simulink model "proportionalNav_withControlSystem"  (R2023b)
settings: Solver=ode4  StartTime=0.0  StopTime=inf  FixedStep=0.001  RelTol=1e-3
model workspace: external: MAT-File C:\proj\simulink_runner.mat (data not in the file)
values from neighbouring files (symbols this model uses):
  Beta = X(5)    [matlab_control_with_comment.m]
  coef_data = struct()    [matlab_control_with_comment.m]
  dry_mass = missile.dry_mass    [matlab_control_with_comment.m]
  fuel_mass = current_fuel_mass + fuel_structure_mass    [matlab_control_with_comment.m]
  g = 9.81    [matlab_control_with_comment.m]
  lref = missile.lref    [matlab_control_with_comment.m]
  q = X_s(11)    [matlab_control_with_comment.m]
  R_Mx = X(6)    [matlab_control_with_comment.m]
  R_Mz = X(7)    [matlab_control_with_comment.m]
  R_Tx = X(1)    [matlab_control_with_comment.m]
  R_Tz = X(2)    [matlab_control_with_comment.m]
  S = missile.S    [matlab_control_with_comment.m]
  t_b = thrust.t_b    [matlab_control_with_comment.m]
  T_total = thrust.T_total    [matlab_control_with_comment.m]
  theta = X(10)    [matlab_control_with_comment.m]
  V_Mx = X(8)    [matlab_control_with_comment.m]
  V_Mz = X(9)    [matlab_control_with_comment.m]
  V_T = target.V_T    [matlab_control_with_comment.m]
  XNP = missile.XNP    [matlab_control_with_comment.m]
  XNT = target.XNT    [matlab_control_with_comment.m]
libraries: simulink_extras x3, simulink x2
settings Model: NumberOfSteps=15  Creator=hamdi  LastModifiedBy=furkan
settings SolverCC: InitialStep=0.001  ZeroCrossAlgorithm=Adaptive

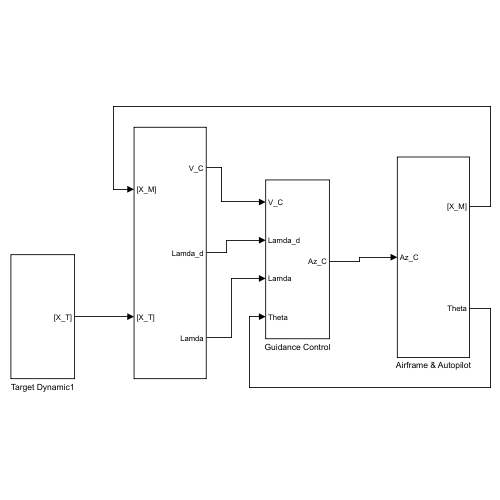
[thumbnail: Simulink's stored preview of the top-level diagram]
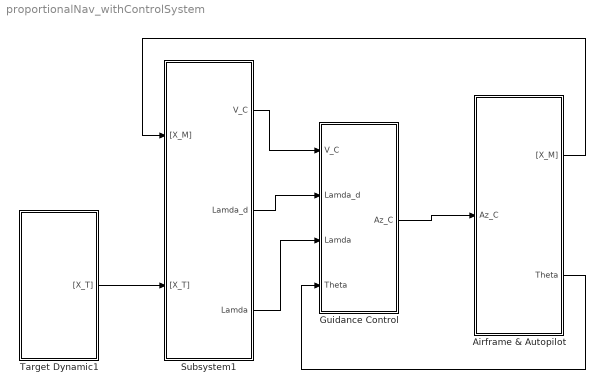
== system proportionalNav_withControlSystem ==
  Airframe & Autopilot : Subsystem
  Guidance Control : Subsystem
  Subsystem1 : Subsystem
  Target Dynamic1 : Subsystem
  wires:
  Subsystem1/2(Lamda_d) -> Guidance Control/2(Lamda_d)
  Target Dynamic1/1("[X_T]") -> Subsystem1/2("[X_T]")
  Subsystem1/1(V_C) -> Guidance Control/1(V_C)
  Subsystem1/3(Lamda) -> Guidance Control/3(Lamda)
  Guidance Control/1(Az_C) -> Airframe & Autopilot/1(Az_C)
  Airframe & Autopilot/1("[X_M]") -> Subsystem1/1("[X_M]")
  Airframe & Autopilot/2(Theta) -> Guidance Control/4(Theta)

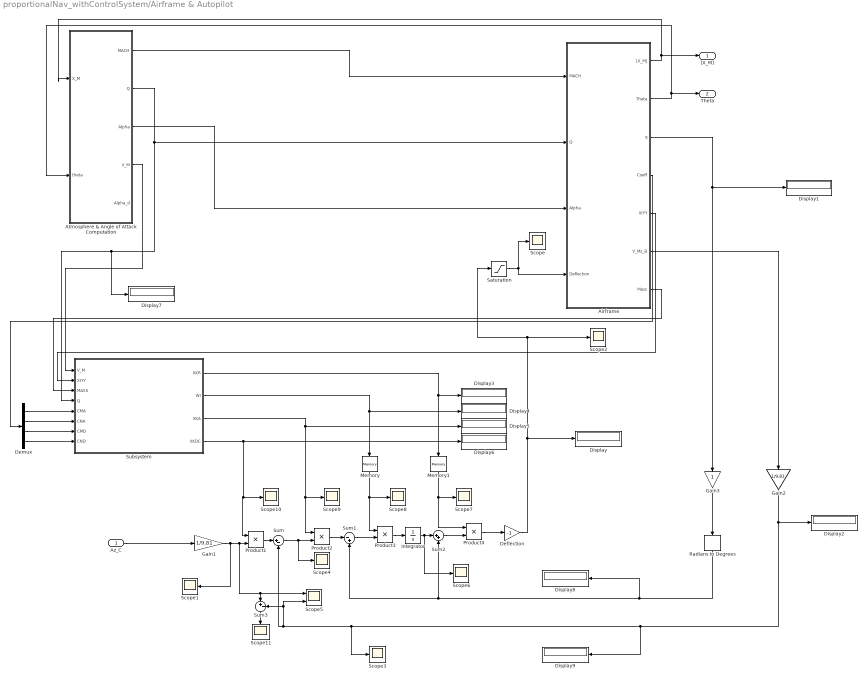
== system proportionalNav_withControlSystem/Airframe & Autopilot ==
  Az_C : Inport
  Airframe : Subsystem
  Atmosphere & Angle of Attack Computation : Subsystem
  Deflection : Gain  Gain=-1
  Demux : Demux
  Display{,1..9} (10 alike) : Display
  Gain1 : Gain  Gain=1/9.81
  Gain2 : Gain  Gain=1/9.81
  Gain3 : Gain
  Integrator : Integrator
  Memory : Memory
  Memory1 : Memory
  Product{1..4} (4 alike) : Product
  Radians to Degrees : simulink_extras/Transformations/Radians to Degrees
  Saturation : Saturate  UpperLimit=19  LowerLimit=-19
  Scope{,1..4,6..11} (11 alike) : Scope
  Scope5 : Scope  NumInputPorts=2
  Subsystem : Subsystem
  Sum : Sum  Inputs=|+-
  Sum1 : Sum  Inputs=|-+
  Sum2 : Sum  Inputs=|++
  Sum3 : Sum  Inputs=|+-
  "[X_M]" : Outport
  Theta : Outport  Port=2
  wires:
  Atmosphere & Angle of Attack Computation/1(MACH) -> Airframe/1(MACH)
  Atmosphere & Angle of Attack Computation/3(Alpha) -> Airframe/3(Alpha)
  Airframe/1("[X_M]") -> "[X_M]"/1, Atmosphere & Angle of Attack Computation/1(X_M)
  Airframe/2(Theta) -> Theta/1, Atmosphere & Angle of Attack Computation/2(theta)
  Product2/1 -> Sum1/1
  Product1/1 -> Sum/1
  Product3/1 -> Integrator/1
  Sum/1 -> Scope4/1, Product2/2
  Sum1/1 -> Product3/2
  Sum2/1 -> Product4/2
  Product4/1 -> Deflection/1
  Subsystem/1(XKR) -> Display3/1, Memory1/1
  Atmosphere & Angle of Attack Computation/4(V_M) -> Subsystem/1(V_M)
  Airframe/4(Coeff) -> Demux/1
  Demux/1 -> Subsystem/5(CMA)
  Demux/2 -> Subsystem/6(CNA)
  Demux/3 -> Subsystem/7(CMD)
  Demux/4 -> Subsystem/8(CND)
  Airframe/5(XIYY) -> Subsystem/2(XIYY)
  Airframe/7(Mass) -> Subsystem/3(MASS)
  Subsystem/2(WI) -> Display4/1, Memory/1
  Memory/1 -> Scope8/1, Product3/1
  Memory1/1 -> Scope7/1, Product4/1
  Integrator/1 -> Scope6/1, Sum2/1
  Gain3/1 -> Radians to Degrees/1
  Deflection/1 -> Saturation/1, Scope2/1, Display/1
  Radians to Degrees/1 -> Display8/1, Sum2/2, Sum1/2
  Atmosphere & Angle of Attack Computation/2(Q) -> Subsystem/4(Q), Display7/1, Airframe/2(Q)
  Airframe/3(q) -> Gain3/1, Display1/1
  Airframe/6(V_Mz_B) -> Gain2/1
  Gain1/1 -> Scope1/1, Sum3/1, Scope5/1, Product1/2
  Saturation/1 -> Scope/1, Airframe/4(Deflection)
  Subsystem/4(XKDC) -> Product1/1, Scope10/1, Display6/1
  Subsystem/3(XKA) -> Scope9/1, Product2/1, Display5/1
  Gain2/1 -> Display2/1, Display9/1, Sum3/2, Scope5/2, Sum/2, Scope3/1
  Sum3/1 -> Scope11/1
  Az_C/1 -> Gain1/1

== system proportionalNav_withControlSystem/Guidance Control ==
  V_C : Inport
  Lamda_d : Inport  Port=2
  Lamda : Inport  Port=3
  Theta : Inport  Port=4
  Cos : Trigonometry  Operator=cos
  Display : Display
  Display1 : Display
  Display2 : Display
  "Effective Navigation Ratio " : Constant  Value=XNP
  Gain1 : Gain  Gain=1/g
  Product : Product
  Product9 : Product  Inputs=3
  Scope1 : Scope
  Subtract : Sum  Inputs=+-
  Az_C : Outport
  wires:
  V_C/1 -> Display/1, Product9/3
  "Effective Navigation Ratio "/1 -> Product9/1
  Lamda_d/1 -> Display1/1, Product9/2
  Product9/1 -> Az_C/1, Product/1, Gain1/1
  Gain1/1 -> Scope1/1, Display2/1
  Theta/1 -> Subtract/1
  Subtract/1 -> Cos/1
  Cos/1 -> Product/2
  Lamda/1 -> Subtract/2

== system proportionalNav_withControlSystem/Subsystem1 ==
  "[X_M]" : Inport
  "[X_T]" : Inport  Port=2
  Compare To Zero : simulink/Logic and Bit Operations/Compare To Zero  relop=<=  OutDataTypeStr=boolean
  Demux : Demux
  Demux1 : Demux
  Display : Display
  Scope : Scope
  Scope2 : Scope
  Stop Simulation : Stop
  Subsystem2 : Subsystem
  V_C : Outport
  Lamda_d : Outport  Port=2
  Lamda : Outport  Port=3
  wires:
  "[X_T]"/1 -> Demux/1
  "[X_M]"/1 -> Demux1/1
  Subsystem2/2(Lamda_d) -> Scope2/1, Lamda_d/1
  Subsystem2/1(V_C) -> Compare To Zero/1, V_C/1, Display/1, Scope/1
  Demux1/1 -> Subsystem2/1(R_Mx)  "R_Mx"
  Demux1/2 -> Subsystem2/2(R_Mz)  "R_Mz"
  Demux1/3 -> Subsystem2/3(V_Mx)  "V_Mx"
  Demux1/4 -> Subsystem2/4(V_Mz)  "V_Mz"
  Demux/1 -> Subsystem2/5(R_Tx)  "R_Tx"
  Demux/2 -> Subsystem2/6(R_Tz)  "R_Tz"
  Demux/3 -> Subsystem2/7(V_Tx)  "V_Tx"
  Demux/4 -> Subsystem2/8(V_Tz)  "V_Tz"
  Compare To Zero/1 -> Stop Simulation/1
  Subsystem2/4(Lamda) -> Lamda/1

== system proportionalNav_withControlSystem/Target Dynamic1 ==
  Mux : Mux
  Subsystem : Subsystem
  "[X_T]" : Outport
  wires:
  Mux/1 -> "[X_T]"/1
  Subsystem/1(R_Tx) -> Mux/1
  Subsystem/2(R_Tz) -> Mux/2
  Subsystem/3(V_Tx) -> Mux/3
  Subsystem/4(V_Tz) -> Mux/4

== system proportionalNav_withControlSystem/Airframe & Autopilot/Airframe ==
  MACH : Inport
  Q : Inport  Port=2
  Alpha : Inport  Port=3
  Deflection : Inport  Port=4
  Acceleration Calculation : Subsystem
  Aerodynamic : Subsystem
  Integration : Subsystem
  Thrust : Subsystem
  "[X_M]" : Outport
  Theta : Outport  Port=2
  q : Outport  Port=3
  Coeff : Outport  Port=4
  XIYY : Outport  Port=5
  V_Mz_B : Outport  Port=6
  Mass : Outport  Port=7
  wires:
  MACH/1 -> Aerodynamic/2(MACH)
  Q/1 -> Aerodynamic/3(Q)
  Alpha/1 -> Aerodynamic/4(Alpha)
  Deflection/1 -> Aerodynamic/5(Deflection)
  Integration/1("[X_M]") -> "[X_M]"/1
  Aerodynamic/1(Aero_X_force) -> Acceleration Calculation/4(Aero_X_force)
  Thrust/1(Thrust) -> Acceleration Calculation/2(Thrust)
  Thrust/3(xcg) -> Aerodynamic/1(XCG)
  Thrust/2(Mass) -> Mass/1, Acceleration Calculation/3(Mass)
  Aerodynamic/3(Moment) -> Integration/3(Moment)
  Acceleration Calculation/1(A_Mx_I) -> Integration/1(A_Mx)
  Acceleration Calculation/2(A_Mz_I) -> Integration/2(A_Mz)
  Thrust/4(Iyy) -> XIYY/1, Integration/4(Iyy)
  Integration/3(q) -> q/1
  Integration/2(Theta) -> Theta/1, Acceleration Calculation/1(Theta)
  Aerodynamic/4(Coeff) -> Coeff/1
  Aerodynamic/2(Aero_Z_force) -> Acceleration Calculation/5(Aero_Z_force)
  Acceleration Calculation/3(Out3) -> V_Mz_B/1

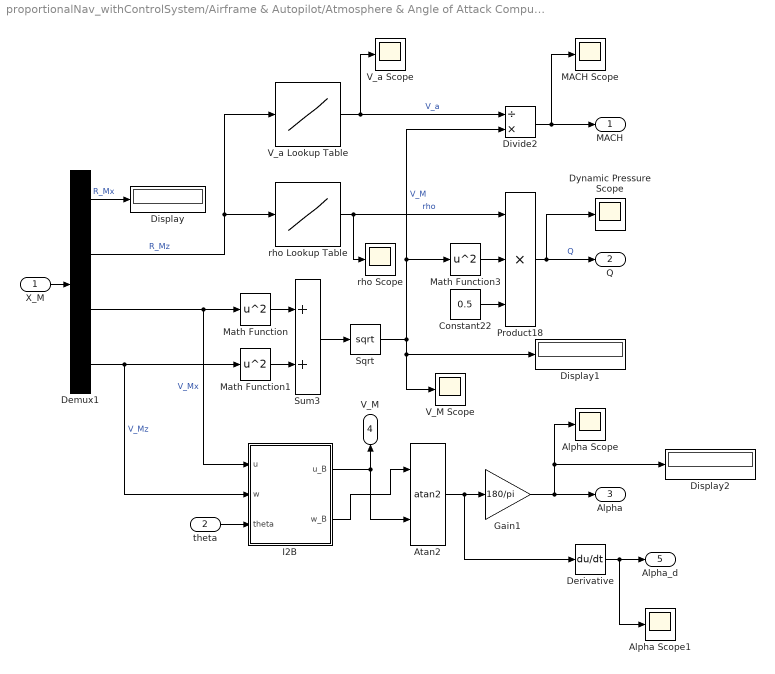
== system proportionalNav_withControlSystem/Airframe & Autopilot/Atmosphere & Angle of Attack Computation ==
  X_M : Inport
  theta : Inport  Port=2
  Alpha Scope : Scope
  Alpha Scope1 : Scope
  Atan2 : Trigonometry  Operator=atan2
  Constant22 : Constant  Value=0.5
  Demux1 : Demux
  Derivative : Derivative
  Display : Display
  Display1 : Display
  Display2 : Display
  Divide2 : Product  Inputs=/*
  Dynamic Pressure Scope : Scope
  Gain1 : Gain  Gain=180/pi
  I2B : MATLAB Function  TreatAsAtomicUnit=on
  MACH Scope : Scope
  Math Function : Math  Operator=square
  Math Function1 : Math  Operator=square
  Math Function3 : Math  Operator=square
  Product18 : Product  Inputs=3
  Sqrt : Sqrt
  Sum3 : Sum
  V_M Scope : Scope
  V_a Lookup Table : Lookup_n-D  NumberOfTableDimensions=1  BreakpointsForDimension1=coef_data.alt_table  Table=coef_data.V_a_table  InternalRulePriority=Speed  RndMeth=Simplest
  V_a Scope : Scope
  rho Lookup Table : Lookup_n-D  NumberOfTableDimensions=1  BreakpointsForDimension1=coef_data.alt_table  Table=coef_data.rho_table  InternalRulePriority=Speed  RndMeth=Simplest
  rho Scope : Scope
  MACH : Outport
  Q : Outport  Port=2
  Alpha : Outport  Port=3
  V_M : Outport  Port=4
  Alpha_d : Outport  Port=5
  wires:
  Demux1/3 -> I2B/1(u), Math Function/1  "V_Mx"
  Demux1/1 -> Display/1  "R_Mx"
  Demux1/2 -> V_a Lookup Table/1, rho Lookup Table/1  "R_Mz"
  Demux1/4 -> Math Function1/1, I2B/2(w)  "V_Mz"
  X_M/1 -> Demux1/1
  Sum3/1 -> Sqrt/1
  Math Function1/1 -> Sum3/2
  Math Function/1 -> Sum3/1
  Math Function3/1 -> Product18/2
  Sqrt/1 -> Display1/1, V_M Scope/1, Divide2/2, Math Function3/1  "V_M"
  Constant22/1 -> Product18/3
  Product18/1 -> Q/1, Dynamic Pressure Scope/1  "Q"
  rho Lookup Table/1 -> rho Scope/1, Product18/1  "rho"
  Divide2/1 -> MACH/1, MACH Scope/1
  I2B/1(u_B) -> V_M/1, Atan2/2
  I2B/2(w_B) -> Atan2/1
  theta/1 -> I2B/3(theta)
  Gain1/1 -> Alpha/1, Display2/1, Alpha Scope/1
  Atan2/1 -> Derivative/1, Gain1/1
  V_a Lookup Table/1 -> V_a Scope/1, Divide2/1  "V_a"
  Derivative/1 -> Alpha Scope1/1, Alpha_d/1

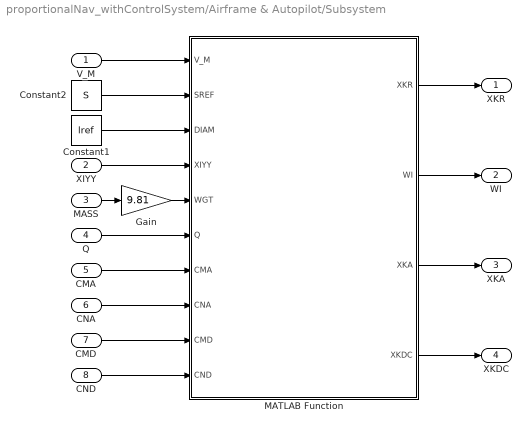
== system proportionalNav_withControlSystem/Airframe & Autopilot/Subsystem ==
  V_M : Inport
  XIYY : Inport  Port=2
  MASS : Inport  Port=3
  Q : Inport  Port=4
  CMA : Inport  Port=5
  CNA : Inport  Port=6
  CMD : Inport  Port=7
  CND : Inport  Port=8
  Constant1 : Constant  Value=lref
  Constant2 : Constant  Value=S
  Gain : Gain  Gain=9.81
  MATLAB Function : MATLAB Function  TreatAsAtomicUnit=on
  XKR : Outport
  WI : Outport  Port=2
  XKA : Outport  Port=3
  XKDC : Outport  Port=4
  wires:
  V_M/1 -> MATLAB Function/1(V_M)
  CMA/1 -> MATLAB Function/7(CMA)
  CNA/1 -> MATLAB Function/8(CNA)
  CMD/1 -> MATLAB Function/9(CMD)
  CND/1 -> MATLAB Function/10(CND)
  MATLAB Function/1(XKR) -> XKR/1
  MATLAB Function/2(WI) -> WI/1
  MATLAB Function/3(XKA) -> XKA/1
  MATLAB Function/4(XKDC) -> XKDC/1
  Q/1 -> MATLAB Function/6(Q)
  Constant2/1 -> MATLAB Function/2(SREF)
  Constant1/1 -> MATLAB Function/3(DIAM)
  XIYY/1 -> MATLAB Function/4(XIYY)
  MASS/1 -> Gain/1
  Gain/1 -> MATLAB Function/5(WGT)

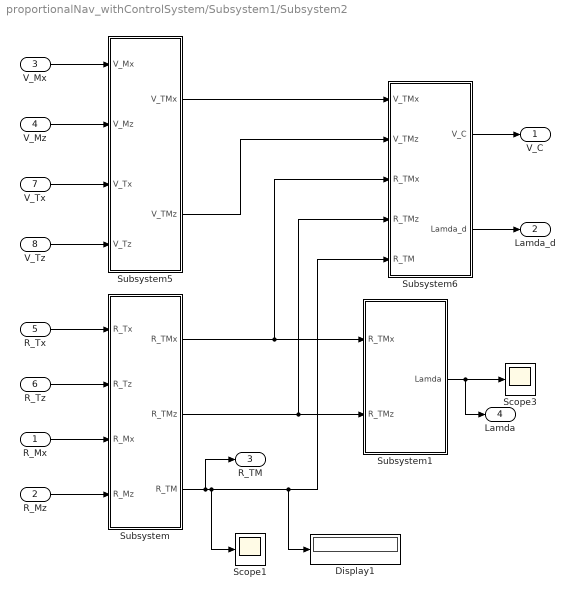
== system proportionalNav_withControlSystem/Subsystem1/Subsystem2 ==
  R_Mx : Inport
  R_Mz : Inport  Port=2
  V_Mx : Inport  Port=3
  V_Mz : Inport  Port=4
  R_Tx : Inport  Port=5
  R_Tz : Inport  Port=6
  V_Tx : Inport  Port=7
  V_Tz : Inport  Port=8
  Display1 : Display
  Scope1 : Scope
  Scope3 : Scope
  Subsystem : Subsystem
  Subsystem1 : Subsystem
  Subsystem5 : Subsystem
  Subsystem6 : Subsystem
  V_C : Outport
  Lamda_d : Outport  Port=2
  R_TM : Outport  Port=3
  Lamda : Outport  Port=4
  wires:
  Subsystem/2(R_TMz) -> Subsystem6/4(R_TMz), Subsystem1/2(R_TMz)
  Subsystem1/1(Lamda) -> Lamda/1, Scope3/1
  Subsystem5/1(V_TMx) -> Subsystem6/1(V_TMx)
  Subsystem/3(R_TM) -> R_TM/1, Subsystem6/5(R_TM), Display1/1, Scope1/1
  V_Tz/1 -> Subsystem5/4(V_Tz)
  Subsystem5/2(V_TMz) -> Subsystem6/2(V_TMz)
  Subsystem/1(R_TMx) -> Subsystem6/3(R_TMx), Subsystem1/1(R_TMx)
  V_Tx/1 -> Subsystem5/3(V_Tx)
  V_Mz/1 -> Subsystem5/2(V_Mz)
  Subsystem6/1(V_C) -> V_C/1
  Subsystem6/2(Lamda_d) -> Lamda_d/1
  V_Mx/1 -> Subsystem5/1(V_Mx)
  R_Mz/1 -> Subsystem/4(R_Mz)
  R_Tx/1 -> Subsystem/1(R_Tx)
  R_Mx/1 -> Subsystem/3(R_Mx)
  R_Tz/1 -> Subsystem/2(R_Tz)

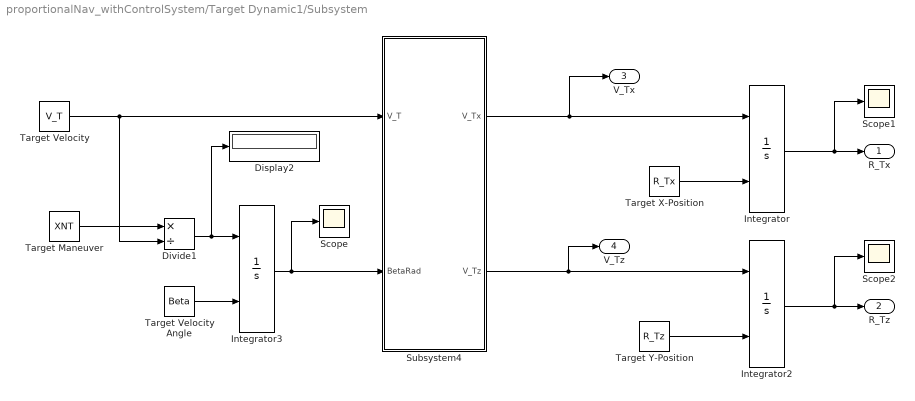
== system proportionalNav_withControlSystem/Target Dynamic1/Subsystem ==
  Display2 : Display
  Divide1 : Product  Inputs=*/
  Integrator : Integrator  InitialConditionSource=external
  Integrator2 : Integrator  InitialConditionSource=external
  Integrator3 : Integrator  InitialConditionSource=external
  Scope : Scope
  Scope1 : Scope
  Scope2 : Scope
  Subsystem4 : Subsystem
  Target Maneuver : Constant  Value=XNT
  Target Velocity : Constant  Value=V_T
  Target Velocity Angle : Constant  Value=Beta
  "Target X-Position " : Constant  Value=R_Tx
  "Target Y-Position " : Constant  Value=R_Tz
  R_Tx : Outport
  R_Tz : Outport  Port=2
  V_Tx : Outport  Port=3
  V_Tz : Outport  Port=4
  wires:
  Target Velocity/1 -> Divide1/2, Subsystem4/1(V_T)
  Subsystem4/2(V_Tz) -> V_Tz/1, Integrator2/1
  Subsystem4/1(V_Tx) -> V_Tx/1, Integrator/1
  Integrator3/1 -> Subsystem4/2(BetaRad), Scope/1
  Integrator/1 -> Scope1/1, R_Tx/1
  "Target Y-Position "/1 -> Integrator2/2
  "Target X-Position "/1 -> Integrator/2
  Integrator2/1 -> R_Tz/1, Scope2/1
  Target Maneuver/1 -> Divide1/1
  Divide1/1 -> Display2/1, Integrator3/1
  Target Velocity Angle/1 -> Integrator3/2

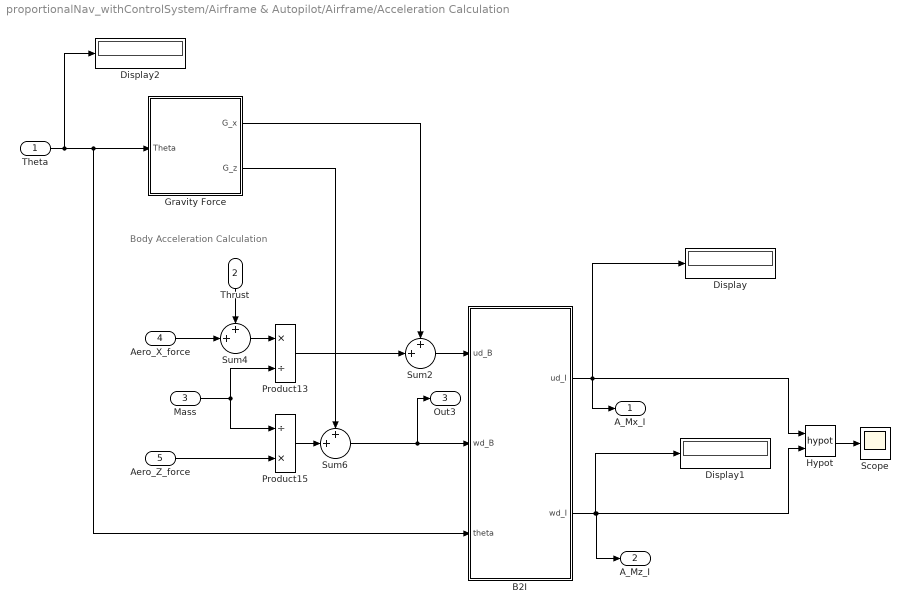
== system proportionalNav_withControlSystem/Airframe & Autopilot/Airframe/Acceleration Calculation ==
  note: Body Acceleration Calculation
  Theta : Inport
  Thrust : Inport  Port=2
  Mass : Inport  Port=3
  Aero_X_force : Inport  Port=4
  Aero_Z_force : Inport  Port=5
  B2I : MATLAB Function  TreatAsAtomicUnit=on
  Display : Display
  Display1 : Display
  Display2 : Display
  Gravity Force : Subsystem
  Hypot : Math  Operator=hypot
  Product13 : Product  Inputs=*/
  Product15 : Product  Inputs=/*
  Scope : Scope
  Sum2 : Sum  Inputs=++|
  Sum4 : Sum  Inputs=++|
  Sum6 : Sum  Inputs=++|
  A_Mx_I : Outport
  A_Mz_I : Outport  Port=2
  Out3 : Outport  Port=3
  wires:
  Theta/1 -> Display2/1, Gravity Force/1(Theta), B2I/3(theta)
  B2I/2(wd_I) -> Display1/1, Hypot/2, A_Mz_I/1
  B2I/1(ud_I) -> Hypot/1, A_Mx_I/1, Display/1
  Sum2/1 -> B2I/1(ud_B)
  Sum4/1 -> Product13/1
  Mass/1 -> Product13/2, Product15/1
  Sum6/1 -> Out3/1, B2I/2(wd_B)
  Aero_X_force/1 -> Sum4/2
  Thrust/1 -> Sum4/1
  Gravity Force/1(G_x) -> Sum2/1
  Aero_Z_force/1 -> Product15/2
  Gravity Force/2(G_z) -> Sum6/1
  Product15/1 -> Sum6/2
  Product13/1 -> Sum2/2
  Hypot/1 -> Scope/1

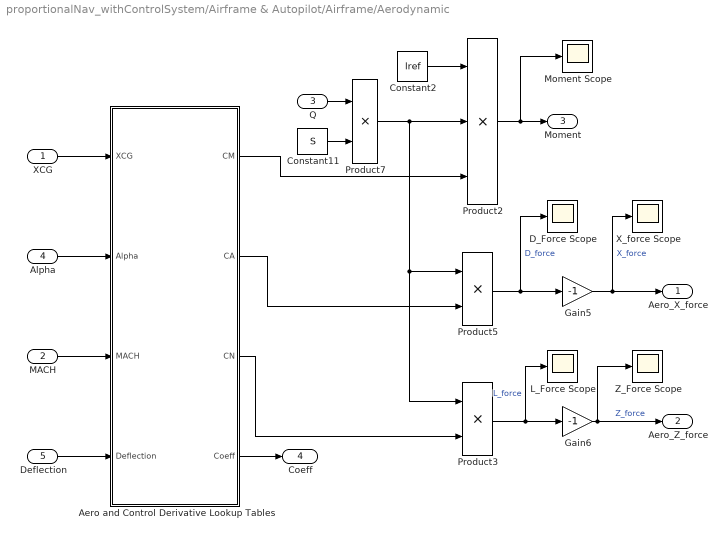
== system proportionalNav_withControlSystem/Airframe & Autopilot/Airframe/Aerodynamic ==
  XCG : Inport
  MACH : Inport  Port=2
  Q : Inport  Port=3
  Alpha : Inport  Port=4
  Deflection : Inport  Port=5
  Aero and Control Derivative Lookup Tables : Subsystem
  Constant11 : Constant  Value=S
  Constant2 : Constant  Value=lref
  D_Force Scope : Scope
  Gain5 : Gain  Gain=-1
  Gain6 : Gain  Gain=-1
  L_Force Scope : Scope
  Moment Scope : Scope
  Product2 : Product  Inputs=3
  Product3 : Product
  Product5 : Product
  Product7 : Product
  X_force Scope : Scope
  Z_Force Scope : Scope
  Aero_X_force : Outport
  Aero_Z_force : Outport  Port=2
  Moment : Outport  Port=3
  Coeff : Outport  Port=4
  wires:
  Constant11/1 -> Product7/2
  Gain6/1 -> Aero_Z_force/1, Z_Force Scope/1  "Z_force"
  Product7/1 -> Product2/2, Product3/1, Product5/1
  Product3/1 -> L_Force Scope/1, Gain6/1  "L_force"
  Product5/1 -> Gain5/1, D_Force Scope/1  "D_force"
  Gain5/1 -> Aero_X_force/1, X_force Scope/1  "X_force"
  XCG/1 -> Aero and Control Derivative Lookup Tables/1(XCG)
  Alpha/1 -> Aero and Control Derivative Lookup Tables/2(Alpha)
  MACH/1 -> Aero and Control Derivative Lookup Tables/3(MACH)
  Aero and Control Derivative Lookup Tables/1(CM) -> Product2/3
  Q/1 -> Product7/1
  Constant2/1 -> Product2/1
  Product2/1 -> Moment Scope/1, Moment/1
  Deflection/1 -> Aero and Control Derivative Lookup Tables/4(Deflection)
  Aero and Control Derivative Lookup Tables/2(CA) -> Product5/2
  Aero and Control Derivative Lookup Tables/3(CN) -> Product3/2
  Aero and Control Derivative Lookup Tables/4(Coeff) -> Coeff/1

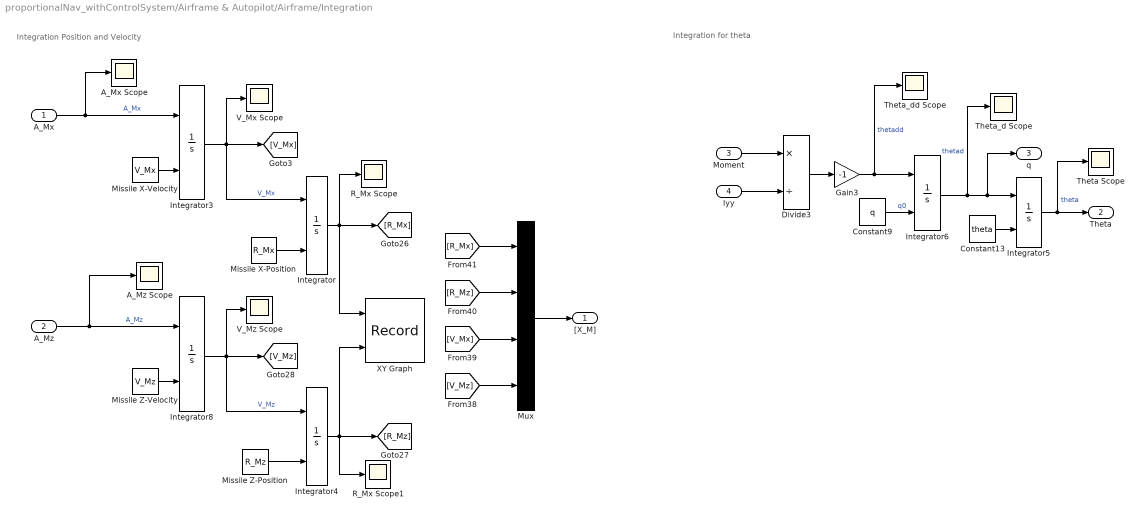
== system proportionalNav_withControlSystem/Airframe & Autopilot/Airframe/Integration ==
  note: Integration for theta
  note: Integration Position and Velocity
  A_Mx : Inport
  A_Mz : Inport  Port=2
  Moment : Inport  Port=3
  Iyy : Inport  Port=4
  A_Mx Scope : Scope
  A_Mz Scope : Scope
  Constant13 : Constant  Value=theta
  Constant9 : Constant  Value=q
  Divide3 : Product  Inputs=*/
  Gain3 : Gain  Gain=-1
  Integrator{,3..6,8} (6 alike) : Integrator  InitialConditionSource=external
  "Missile X-Position " : Constant  Value=R_Mx
  Missile X-Velocity : Constant  Value=V_Mx
  Missile Z-Position : Constant  Value=R_Mz
  Missile Z-Velocity : Constant  Value=V_Mz
  Mux : Mux
  R_Mx Scope : Scope
  R_Mx Scope1 : Scope
  Theta Scope : Scope
  Theta_d Scope : Scope
  Theta_dd Scope : Scope
  V_Mx Scope : Scope
  V_Mz Scope : Scope
  XY Graph : Record  FileSettingsInternal="{\"entries\":[{\"content\":{\"excelSettings\":{\"content\":{},\"type\":\"Streamout.ExcelSettings\"}},\"type\":\"Streamout.FileSettingStorage\",\"uuid\":\"\"}],\"packageUris\":[\"http:\\/\\/schema.mathworks.com\\/mf0\\/streamout_blocks\\/R2020a\"],\"version\":\"1.0\"}"  Layout=[1 1]  SignalsInternal="{\"entries\":[{\"content\":{\"signals\":[{\"content\":{\"blockPath\":[],\"dimensions\":[1],\"domain\":\"\",\"lineColor\":\"#a2142f\",\"plots\":[ 1 ],\"port\":1,\"sid\":[\"\"],\"signalID\":1,\"signalName\":\"Integrator\"},\"type\":\"RecordBlkView.Signal\",\"uuid\":\"\"},{\"content\":{\"blockPath\":[],\"dimensions\":[1],\"domain\":\"\",\"lineColor\":\"#139fff\",\"plots\":[ 1 ],\"port\":2,\"sid\":[\"\"],\"signalID\":2,\"signalName\":\"Integrator4\"},\"type\":\"RecordBlkView.Signal\",\"uuid\":\"\"}]},\"type\":\"RecordBlkView.InputSignals\",\"uuid\":\"\"}],\"packageUris\":[\"http:\\/\\/schema.mathworks.com\\/mf0\\/streamout_blocks\\/R2020a\"],\"version\":\"1.0\"}"  VisualizationBindings="{\"xyplotplugin\":{\"info\":[{\"series\":[{\"bindingParametersList\":[{\"parameter\":\"X-Axis\",\"signalID\":1,\"signalName\":\"Integrator\"},{\"parameter\":\"Y-Axis\",\"signalID\":2,\"signalName\":\"Integrator4\"}],\"seriesID\":0}],\"subplotID\":1}]}}"  CompatibilityTag=XY
  "[X_M]" : Outport
  Theta : Outport  Port=2
  q : Outport  Port=3
  wires:
  Constant13/1 -> Integrator5/2
  Integrator6/1 -> Theta_d Scope/1, q/1, Integrator5/1  "thetad"
  Constant9/1 -> Integrator6/2  "q0"
  Divide3/1 -> Gain3/1
  Integrator5/1 -> Theta/1, Theta Scope/1  "theta"
  Gain3/1 -> Theta_dd Scope/1, Integrator6/1  "thetadd"
  [R_Mz] -> Mux/2
  Missile Z-Velocity/1 -> Integrator8/2
  [V_Mz] -> Mux/4
  Missile Z-Position/1 -> Integrator4/2
  Integrator4/1 -> R_Mx Scope1/1, XY Graph/2, [R_Mz]
  Integrator3/1 -> [V_Mx], Integrator/1, V_Mx Scope/1  "V_Mx"
  [R_Mx] -> Mux/1
  Missile X-Velocity/1 -> Integrator3/2
  Integrator/1 -> XY Graph/1, [R_Mx], R_Mx Scope/1
  A_Mz/1 -> Integrator8/1, A_Mz Scope/1  "A_Mz"
  [V_Mx] -> Mux/3
  "Missile X-Position "/1 -> Integrator/2
  Integrator8/1 -> [V_Mz], Integrator4/1, V_Mz Scope/1  "V_Mz"
  Iyy/1 -> Divide3/2
  Moment/1 -> Divide3/1
  A_Mx/1 -> A_Mx Scope/1, Integrator3/1  "A_Mx"
  Mux/1 -> "[X_M]"/1

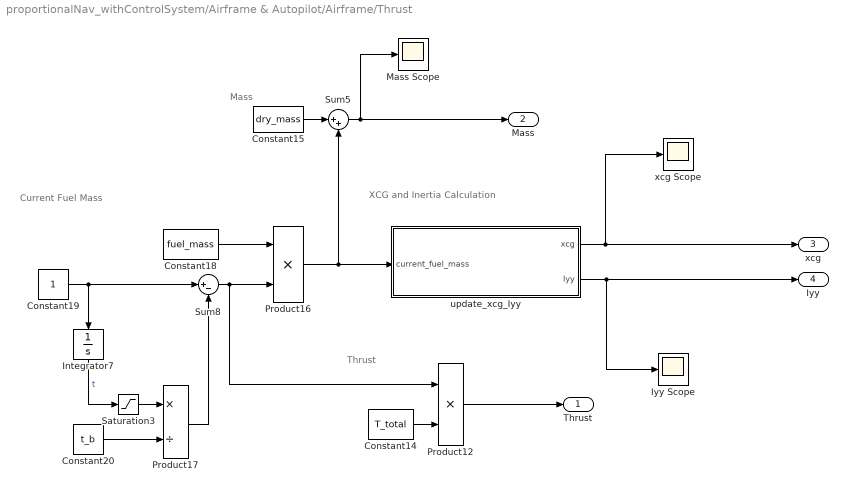
== system proportionalNav_withControlSystem/Airframe & Autopilot/Airframe/Thrust ==
  note: XCG and Inertia Calculation
  note: Mass
  note: Current Fuel Mass
  note: Thrust
  Constant14 : Constant  Value=T_total
  Constant15 : Constant  Value=dry_mass
  Constant18 : Constant  Value=fuel_mass
  Constant19 : Constant
  Constant20 : Constant  Value=t_b
  Integrator7 : Integrator
  Iyy Scope : Scope
  Mass Scope : Scope
  Product12 : Product
  Product16 : Product
  Product17 : Product  Inputs=*/
  Saturation3 : Saturate  UpperLimit=t_b  LowerLimit=0
  Sum5 : Sum  Inputs=|++
  Sum8 : Sum  Inputs=|+-
  update_xcg_Iyy : MATLAB Function  TreatAsAtomicUnit=on
  xcg Scope : Scope
  Thrust : Outport
  Mass : Outport  Port=2
  xcg : Outport  Port=3
  Iyy : Outport  Port=4
  wires:
  Constant15/1 -> Sum5/1
  Integrator7/1 -> Saturation3/1  "t"
  Saturation3/1 -> Product17/1
  Product17/1 -> Sum8/2
  Constant20/1 -> Product17/2
  Constant19/1 -> Integrator7/1, Sum8/1
  Sum8/1 -> Product12/1, Product16/2
  Constant18/1 -> Product16/1
  Product16/1 -> Sum5/2, update_xcg_Iyy/1(current_fuel_mass)
  Constant14/1 -> Product12/2
  update_xcg_Iyy/1(xcg) -> xcg Scope/1, xcg/1
  update_xcg_Iyy/2(Iyy) -> Iyy/1, Iyy Scope/1
  Sum5/1 -> Mass/1, Mass Scope/1
  Product12/1 -> Thrust/1

== system proportionalNav_withControlSystem/Subsystem1/Subsystem2/Subsystem ==
  R_Tx : Inport
  R_Tz : Inport  Port=2
  R_Mx : Inport  Port=3
  R_Mz : Inport  Port=4
  Add1 : Sum
  Compare To Constant : simulink/Logic and Bit Operations/Compare To Constant  relop=<=  const=0  OutDataTypeStr=boolean
  Constant : Constant  Value=2
  Power : Math  Operator=pow
  Power1 : Math  Operator=pow
  Sqrt : Sqrt
  Stop Simulation : Stop
  Subtract : Sum  Inputs=+-
  Subtract1 : Sum  Inputs=+-
  R_TMx : Outport
  R_TMz : Outport  Port=2
  R_TM : Outport  Port=3
  wires:
  Subtract1/1 -> Power1/1, R_TMz/1
  Constant/1 -> Power1/2, Power/2
  Power1/1 -> Add1/2
  Add1/1 -> Sqrt/1
  Power/1 -> Add1/1
  Subtract/1 -> Power/1, R_TMx/1
  R_Tz/1 -> Subtract1/1
  R_Mz/1 -> Subtract1/2
  R_Mx/1 -> Subtract/2
  R_Tx/1 -> Subtract/1
  Sqrt/1 -> Compare To Constant/1, R_TM/1
  Compare To Constant/1 -> Stop Simulation/1

== system proportionalNav_withControlSystem/Subsystem1/Subsystem2/Subsystem1 ==
  R_TMx : Inport
  R_TMz : Inport  Port=2
  Atan2 : Trigonometry  Operator=atan2
  Lamda : Outport
  wires:
  Atan2/1 -> Lamda/1
  R_TMx/1 -> Atan2/2
  R_TMz/1 -> Atan2/1

== system proportionalNav_withControlSystem/Subsystem1/Subsystem2/Subsystem5 ==
  V_Mx : Inport
  V_Mz : Inport  Port=2
  V_Tx : Inport  Port=3
  V_Tz : Inport  Port=4
  Subtract2 : Sum  Inputs=+-
  Subtract3 : Sum  Inputs=+-
  V_TMx : Outport
  V_TMz : Outport  Port=2
  wires:
  V_Tz/1 -> Subtract3/1
  V_Mx/1 -> Subtract2/2
  V_Mz/1 -> Subtract3/2
  V_Tx/1 -> Subtract2/1
  Subtract2/1 -> V_TMx/1
  Subtract3/1 -> V_TMz/1

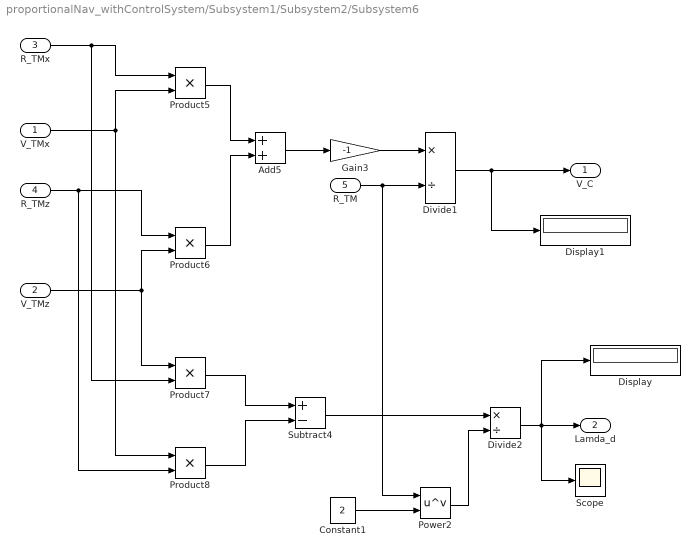
== system proportionalNav_withControlSystem/Subsystem1/Subsystem2/Subsystem6 ==
  V_TMx : Inport
  V_TMz : Inport  Port=2
  R_TMx : Inport  Port=3
  R_TMz : Inport  Port=4
  R_TM : Inport  Port=5
  Add5 : Sum
  Constant1 : Constant  Value=2
  Display : Display
  Display1 : Display
  Divide1 : Product  Inputs=*/
  Divide2 : Product  Inputs=*/
  Gain3 : Gain  Gain=-1
  Power2 : Math  Operator=pow
  Product{5..8} (4 alike) : Product
  Scope : Scope
  Subtract4 : Sum  Inputs=+-
  V_C : Outport
  Lamda_d : Outport  Port=2
  wires:
  R_TMz/1 -> Product6/1, Product8/2
  Add5/1 -> Gain3/1
  R_TM/1 -> Power2/1, Divide1/2
  R_TMx/1 -> Product5/1, Product7/2
  V_TMx/1 -> Product8/1, Product5/2
  Product6/1 -> Add5/2
  V_TMz/1 -> Product7/1, Product6/2
  Product5/1 -> Add5/1
  Subtract4/1 -> Divide2/1
  Power2/1 -> Divide2/2
  Product8/1 -> Subtract4/2
  Divide2/1 -> Scope/1, Display/1, Lamda_d/1
  Product7/1 -> Subtract4/1
  Constant1/1 -> Power2/2
  Divide1/1 -> Display1/1, V_C/1
  Gain3/1 -> Divide1/1

== system proportionalNav_withControlSystem/Target Dynamic1/Subsystem/Subsystem4 ==
  note: Input 1: V_T % Velocity of the target (ft/s)
      | Input 2: Beta % Angle of the target velocity (rad)
  note: Output 1: V_Tx = -V_T*cos(BetaRad) % Target velocity X-Component (ft/s)
      | Output 2: V_Ty = V_T*sin(BetaRad) % Target velocity Y-Component (ft/s)
  V_T : Inport
  BetaRad : Inport  Port=2
  Cos : Trigonometry  Operator=cos
  Gain1 : Gain  Gain=-1
  Product : Product
  Product1 : Product
  Scope1 : Scope
  Scope2 : Scope
  Sin : Trigonometry
  V_Tx : Outport
  V_Tz : Outport  Port=2
  wires:
  V_T/1 -> Product1/1, Gain1/1
  Gain1/1 -> Product/2
  Cos/1 -> Product/1
  BetaRad/1 -> Sin/1, Cos/1
  Sin/1 -> Product1/2
  Product/1 -> Scope1/1, V_Tx/1
  Product1/1 -> Scope2/1, V_Tz/1

== system proportionalNav_withControlSystem/Airframe & Autopilot/Airframe/Acceleration Calculation/Gravity Force ==
  Theta : Inport
  Constant16 : Constant  Value=g
  Constant17 : Constant  Value=g
  Gain1 : Gain  Gain=-1
  Gain8 : Gain  Gain=-1
  Product14 : Product
  Product8 : Product
  cos : Trigonometry  Operator=cos
  sin : Trigonometry
  G_x : Outport
  G_z : Outport  Port=2
  wires:
  Product8/1 -> Gain8/1
  Theta/1 -> cos/1, sin/1
  sin/1 -> Product14/2
  Gain8/1 -> G_z/1  "q"
  Constant17/1 -> Product8/2
  Constant16/1 -> Product14/1
  Gain1/1 -> G_x/1  "q"
  cos/1 -> Product8/1
  Product14/1 -> Gain1/1

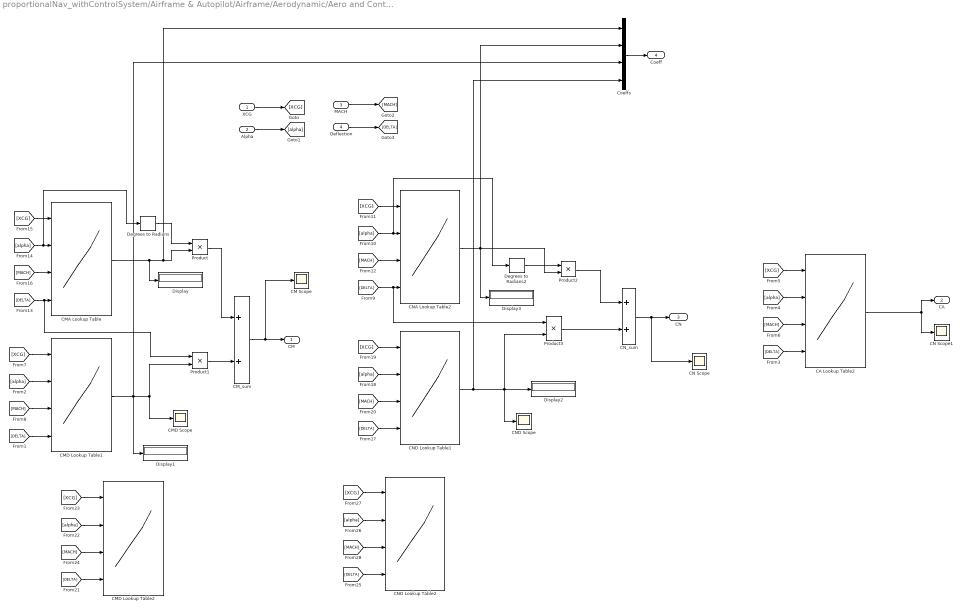
== system proportionalNav_withControlSystem/Airframe & Autopilot/Airframe/Aerodynamic/Aero and Control Derivative Lookup Tables ==
  XCG : Inport
  Alpha : Inport  Port=2
  MACH : Inport  Port=3
  Deflection : Inport  Port=4
  CA Lookup Table2 : Lookup_n-D  NumberOfTableDimensions=4  BreakpointsForDimension1=coef_data.XCG_grid  BreakpointsForDimension2=coef_data.ALPHA_grid  BreakpointsForDimension3=coef_data.MACH_grid  BreakpointsForDimension4=coef_data.DELTA_grid  Table=coef_data.CA_data  InternalRulePriority=Speed  RndMeth=Simplest
      settings: InputPortMap=u0,u1,u2,u3
  CM Scope : Scope
  CMA Lookup Table : Lookup_n-D  NumberOfTableDimensions=4  BreakpointsForDimension1=coef_data.XCG_grid  BreakpointsForDimension2=coef_data.ALPHA_grid  BreakpointsForDimension3=coef_data.MACH_grid  BreakpointsForDimension4=coef_data.DELTA_grid  Table=coef_data.CMA_data  InternalRulePriority=Speed  RndMeth=Simplest
      settings: InputPortMap=u0,u1,u2,u3
  CMD Lookup Table1 : Lookup_n-D  NumberOfTableDimensions=4  BreakpointsForDimension1=coef_data.XCG_grid  BreakpointsForDimension2=coef_data.ALPHA_grid  BreakpointsForDimension3=coef_data.MACH_grid  BreakpointsForDimension4=coef_data.DELTA_grid  Table=coef_data.CMD_data  InternalRulePriority=Speed  RndMeth=Simplest
      settings: InputPortMap=u0,u1,u2,u3
  CMD Lookup Table2 : Lookup_n-D  NumberOfTableDimensions=4  BreakpointsForDimension1=coef_data.XCG_grid  BreakpointsForDimension2=coef_data.ALPHA_grid  BreakpointsForDimension3=coef_data.MACH_grid  BreakpointsForDimension4=coef_data.DELTA_grid  Table=coef_data.CM_data  InternalRulePriority=Speed  RndMeth=Simplest
      settings: InputPortMap=u0,u1,u2,u3
  CMD Scope : Scope
  CM_sum : Sum  InputSameDT=on  SaturateOnIntegerOverflow=on  OutDataTypeStr=Inherit: Same as first input
  CN Scope : Scope
  CN Scope1 : Scope
  CNA Lookup Table2 : Lookup_n-D  NumberOfTableDimensions=4  BreakpointsForDimension1=coef_data.XCG_grid  BreakpointsForDimension2=coef_data.ALPHA_grid  BreakpointsForDimension3=coef_data.MACH_grid  BreakpointsForDimension4=coef_data.DELTA_grid  Table=coef_data.CNA_data  InternalRulePriority=Speed  RndMeth=Simplest
      settings: InputPortMap=u0,u1,u2,u3
  CND Lookup Table1 : Lookup_n-D  NumberOfTableDimensions=4  BreakpointsForDimension1=coef_data.XCG_grid  BreakpointsForDimension2=coef_data.ALPHA_grid  BreakpointsForDimension3=coef_data.MACH_grid  BreakpointsForDimension4=coef_data.DELTA_grid  Table=coef_data.CND_data  InternalRulePriority=Speed  RndMeth=Simplest
      settings: InputPortMap=u0,u1,u2,u3
  CND Lookup Table2 : Lookup_n-D  NumberOfTableDimensions=4  BreakpointsForDimension1=coef_data.XCG_grid  BreakpointsForDimension2=coef_data.ALPHA_grid  BreakpointsForDimension3=coef_data.MACH_grid  BreakpointsForDimension4=coef_data.DELTA_grid  Table=coef_data.CN_data  InternalRulePriority=Speed  RndMeth=Simplest
      settings: InputPortMap=u0,u1,u2,u3
  CND Scope : Scope
  CN_sum : Sum  InputSameDT=on  SaturateOnIntegerOverflow=on  OutDataTypeStr=Inherit: Same as first input
  Coeffs : Mux
  Degrees to Radians : simulink_extras/Transformations/Degrees to Radians
  Degrees to Radians2 : simulink_extras/Transformations/Degrees to Radians
  Display{,1..3} (4 alike) : Display
  Product{,1..3} (4 alike) : Product
  CM : Outport
  CA : Outport  Port=2
  CN : Outport  Port=3
  Coeff : Outport  Port=4
  wires:
  XCG/1 -> [XCG]
  Alpha/1 -> [alpha]
  MACH/1 -> [MACH]
  Deflection/1 -> [DELTA]
  [alpha] -> CND Lookup Table1/2
  [alpha] -> Degrees to Radians/1, CMA Lookup Table/2
  [DELTA] -> CMD Lookup Table1/4
  [MACH] -> CMD Lookup Table1/3
  [DELTA] -> CND Lookup Table1/4
  [alpha] -> CA Lookup Table2/2
  CMA Lookup Table/1 -> Display/1, Coeffs/1, Product/2
  [MACH] -> CA Lookup Table2/3
  [DELTA] -> Product1/1, CMA Lookup Table/4
  [XCG] -> CA Lookup Table2/1
  [XCG] -> CMD Lookup Table1/1
  [MACH] -> CNA Lookup Table2/3
  [alpha] -> Degrees to Radians2/1, CNA Lookup Table2/2
  [XCG] -> CND Lookup Table1/1
  [MACH] -> CND Lookup Table1/3
  [XCG] -> CMA Lookup Table/1
  [MACH] -> CMA Lookup Table/3
  [DELTA] -> CA Lookup Table2/4
  [XCG] -> CNA Lookup Table2/1
  [alpha] -> CMD Lookup Table1/2
  Degrees to Radians/1 -> Product/1
  Product/1 -> CM_sum/1
  Degrees to Radians2/1 -> Product2/1
  Product2/1 -> CN_sum/1
  [DELTA] -> Product3/1, CNA Lookup Table2/4
  Product3/1 -> CN_sum/2
  CA Lookup Table2/1 -> CA/1, CN Scope1/1
  [MACH] -> CMD Lookup Table2/3
  [alpha] -> CMD Lookup Table2/2
  [DELTA] -> CMD Lookup Table2/4
  [XCG] -> CMD Lookup Table2/1
  [XCG] -> CND Lookup Table2/1
  [alpha] -> CND Lookup Table2/2
  [DELTA] -> CND Lookup Table2/4
  [MACH] -> CND Lookup Table2/3
  Product1/1 -> CM_sum/2
  Coeffs/1 -> Coeff/1
  CMD Lookup Table1/1 -> Display1/1, Coeffs/3, CMD Scope/1, Product1/2
  CND Lookup Table1/1 -> Display2/1, Product3/2, CND Scope/1, Coeffs/4
  CNA Lookup Table2/1 -> Display3/1, Coeffs/2, Product2/2
  CM_sum/1 -> CM Scope/1, CM/1
  CN_sum/1 -> CN Scope/1, CN/1

== matlab function proportionalNav_withControlSystem/Airframe & Autopilot/Subsystem/MATLAB Function ==
  data: XKR output; WI output; XKA output; V_M input; SREF input; DIAM input; XIYY input; WGT input; Q input; CMA input; XKDC output; CNA input; CMD input; CND input
function [XKR, WI, XKA, XKDC] = controller_gains(V_M, SREF, DIAM, XIYY, WGT, Q, CMA, CNA, CMD, CND)
    % Initialize outputs
    XKR = 0.0; %#ok<NASGU>
    WI = 0.0; %#ok<NASGU>
    XKA = 0.0; %#ok<NASGU>
    XKDC = 0.0; %#ok<NASGU>

    % Useful Constants
    r2d = 180/pi;                             % Conversion Rad to Deg
    d2r = pi/180;
    g = 9.81;                                 % Gravitational constant (m/s^2)

    % Align coefficient units
    CMD = CMD / d2r;
    CND = CND / d2r;

    % Control Systems Parameters
    WCR = 50;                                % Crossover Frequency (rad/s)
    ZETA = 0.7;                               % Actuator damping
    TAU = 0.3;                                % Time constant (s)

    % Coefficients
    XMA = Q*SREF*DIAM*CMA/XIYY;               % M_∝ (1/s^2)
    XMD = Q*SREF*DIAM*CMD/XIYY;               % M_δ (1/s^2)
    ZA = -g*Q*SREF*CNA/((WGT)*V_M);             % Z_∝ (1/s)
    ZD = -g*Q*SREF*CND/((WGT)*V_M);             % Z_δ (1/s)
    
    % Math
    WZ = sqrt((XMA*ZD-ZA*XMD)/ZD);            % ω_z:  Airframe Zero (rad/s)
    WAF = sqrt(-XMA);                         % ω_AF: Airframe Natural Frequency (rad/s)
    ZAF = 0.5*WAF*ZA/XMA;                     % ξ_AF: Airframe Damping
    XK1 = -V_M*(XMA*ZD-XMD*ZA)/(g*r2d*XMA);   % Gain K1: Aerodynamic acceleration gain (g/deg)
    % XK2 = XK1;                              % Gain K2: Aerodynamic acceleration gain (g/deg)
    TA = XMD/(XMA*ZD-XMD*ZA);                 % T_∝: Turning rate time constant (s)
    XK3 = r2d*g*XK1/V_M;                      % Gain K3: Aerodynamic body rate gain (1/s)
    
    W = (TAU*WCR*(1+2.*ZAF*WAF/WCR)-1)/(2*ZETA*TAU); % Autopilot design parameter 
    W0 = W/sqrt(TAU*WCR);                            % Normalized frequency for autopilot 
    Z0 = 0.5*W0*(2*ZETA/W+TAU-WAF^2/(W0*W0*WCR));    % Damping for autopilot 
    XKC = (-W0^2/WZ^2-1.+2.*Z0*W0*TA)/(1.-2.*Z0*W0*TA+W0*W0*TA*TA);  % Feedback gain for autopilot 
    XKA = XK3/(XK1*XKC);                      % Accelerometer autopilot gain
    XK0 = -W*W/(TAU*WAF*WAF);                 % Open-loop gain for autopilot 
    XK = XK0/(XK1*(1+XKC));                   % Closed-loop gain for autopilot 
    WI = XKC*TA*W0*W0/(1+XKC+W0^2/WZ^2);      % Integrator frequency for autopilot
    XKR = XK/(XKA*WI);                        % Rate gyro gain for autopilot
    XKDC = 1 + g*r2d / (XKA*V_M);             % Steady-state gain for autopilot
end

== matlab function proportionalNav_withControlSystem/Airframe & Autopilot/Atmosphere & Angle of Attack Computation/I2B ==
  data: u input; u_B output; w_B output; w input; theta input
    % ==== Transformation ====
    function [u_B, w_B] = transform(u, w, theta)
            u_B =  cos(theta) * u + sin(theta) * w;
            w_B = -sin(theta) * u + cos(theta) * w;
    end

== matlab function proportionalNav_withControlSystem/Airframe & Autopilot/Airframe/Thrust/update_xcg_Iyy ==
  data: current_fuel_mass input; xcg output; Iyy output
function [xcg, Iyy] = update_xcg_Iyy(current_fuel_mass)
    in2m = 0.0254;
    lb_in3_to_kg_m3 = 27679.9;

    diameter = 12 * in2m;
    r = diameter / 2;

    % Nose
    nose_L = 36 * in2m;
    nose_rho = 0.1 * lb_in3_to_kg_m3;
    nose_xcg = (2/3) * nose_L;
    nose_volume = (1/3) * pi * r^2 * nose_L;
    nose_mass = nose_volume * nose_rho;
    Iyy_nose = (3/20) * nose_mass * r^2;

    % GNC
    GNC_L = 36 * in2m;
    GNC_rho = 0.1 * lb_in3_to_kg_m3;
    GNC_xcg = GNC_L/2 + nose_xcg;
    GNC_volume = pi * r^2 * GNC_L;
    GNC_mass = GNC_volume * GNC_rho;
    Iyy_GNC = (1/12) * GNC_mass * (3*r^2 + GNC_L^2);

    % Warhead
    warhead_L = 72 * in2m;
    warhead_rho = 0.13 * lb_in3_to_kg_m3;
    warhead_xcg = warhead_L/2 + GNC_xcg;
    warhead_volume = pi * r^2 * warhead_L;
    warhead_mass = warhead_volume * warhead_rho;
    Iyy_warhead = (1/12) * warhead_mass * (3*r^2 + warhead_L^2);

    % Fuel
    fuel_L = 96 * in2m;
    structure_rho = 0.06 * lb_in3_to_kg_m3;
    fuel_volume = pi * r^2 * fuel_L;
    fuel_structure_mass = fuel_volume * structure_rho;
    fuel_mass = current_fuel_mass + fuel_structure_mass;
    fuel_xcg = fuel_L/2 + warhead_xcg;
    Iyy_fuel = (1/12) * fuel_mass * (3*r^2 + fuel_L^2);

    % Fins
    rho_fin = 0.12 * lb_in3_to_kg_m3;
    fin_thickness = 0.2 * in2m;

    front_chord = 72 * in2m;
    front_span = 24 * in2m;
    front_root = 84 * in2m;
    front_area = 0.5 * front_chord * front_span;
    front_volume = front_area * fin_thickness;
    front_mass = front_volume * rho_fin * 4;
    front_xcg = front_root + front_chord / 3;
    Iyy_front_fins = 4 * (1/36) * (front_mass / 4) * (front_chord^2 + front_span^2);

    rear_chord = 24 * in2m;
    rear_span = 24 * in2m;
    rear_root = 216 * in2m;
    rear_area = 0.5 * rear_chord * rear_span;
    rear_volume = rear_area * fin_thickness;
    rear_mass = rear_volume * rho_fin * 4;
    rear_xcg = rear_root + rear_chord / 3;
    Iyy_rear_fins = 4 * (1/36) * (rear_mass / 4) * (rear_chord^2 + rear_span^2);

    % Mass
    mass = nose_mass + GNC_mass + warhead_mass + front_mass + rear_mass + fuel_mass;

    % xcg
    xcg = (nose_mass * nose_xcg + GNC_mass * GNC_xcg + warhead_mass * warhead_xcg + ...
           fuel_mass * fuel_xcg + front_mass * front_xcg + rear_mass * rear_xcg) / mass;

    % Distances
    d_nose = abs(nose_xcg - xcg);
    d_GNC = abs(GNC_xcg - xcg);
    d_warhead = abs(warhead_xcg - xcg);
    d_fuel = abs(fuel_xcg - xcg);
    d_front = abs(front_xcg - xcg);
    d_rear = abs(rear_xcg - xcg);

    Iyy = ...
        Iyy_nose + nose_mass * d_nose^2 + ...
        Iyy_GNC + GNC_mass * d_GNC^2 + ...
        Iyy_warhead + warhead_mass * d_warhead^2 + ...
        Iyy_fuel + fuel_mass * d_fuel^2 + ...
        Iyy_front_fins + front_mass * d_front^2 + ...
        Iyy_rear_fins + rear_mass * d_rear^2;
end

== matlab function proportionalNav_withControlSystem/Airframe & Autopilot/Airframe/Acceleration Calculation/B2I ==
  data: ud_B input; ud_I output; wd_I output; wd_B input; theta input
    % ==== Transformation ====
    function [ud_I, wd_I] = transform(ud_B, wd_B, theta)
            ud_I =  cos(theta) * ud_B - sin(theta) * wd_B;
            wd_I =  sin(theta) * ud_B + cos(theta) * wd_B;
    end
